simulink model "solar_collector_model_2019b"  (R2019b)
settings: Solver=VariableStepAuto  StartTime=0.0  StopTime=8760  FixedStep=1  RelTol=1e-3
values from neighbouring files (symbols this model uses):
  a1 = Ac*eta/C    (= 0.000575964912281)    [solar_collector_model_init.m]
  a2 = -UL_1*Ac/C    (= -0.00290974481659)    [solar_collector_model_init.m]
  a3 = -UL_2*Ac/C    (= -7.48006379585e-06)    [solar_collector_model_init.m]
  a4 = V^-1    (= 333.333333333)    [solar_collector_model_init.m]
  a5 = -a4    (= -333.333333333)    [solar_collector_model_init.m]
libraries: simulink x1
settings Model: Creator=Mariana  LastModifiedBy=admin

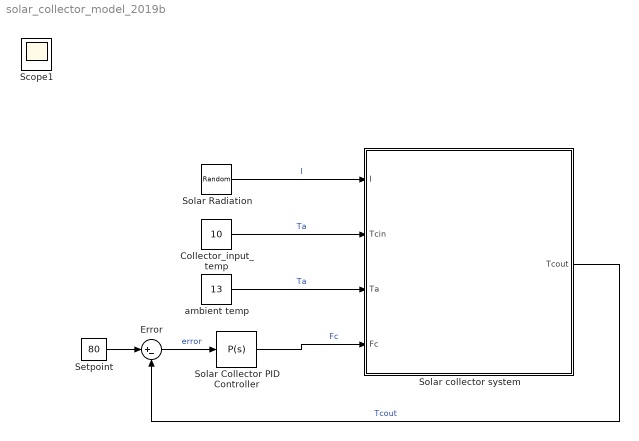
== system solar_collector_model_2019b ==
  "Collector_input_temp " : Constant  Value=10
  Error : Sum  Inputs=|+-
  Setpoint : Constant  Value=80
  Solar Collector PID Controller : simulink/Continuous/PID Controller  Controller=P  Form=Parallel  TimeDomain=Continuous-time  SampleTime=-1  IntegratorMethod=Forward Euler  FilterMethod=Forward Euler  ControllerParametersSource=internal  P=-0.0002  I=1.2  D=0.01  UseFilter=on  N=100  TunerSelectOption=Transfer Function Based (PID Tuner App)  ZeroCross=off  InitialConditionSource=internal  InitialConditionForIntegrator=0  InitialConditionForFilter=0  DifferentiatorICPrevScaledInput=0  ExternalReset=none  TrackingMode=off  Kt=1  LimitOutput=on  UpperSaturationLimit=0.00015  LowerSaturationLimit=0  LinearizeAsGain=on  AntiWindupMode=none  Kb=1  POutMin=[]  POutMax=[]  IOutMin=[]  IOutMax=[]  DOutMin=[]  DOutMax=[]  NOutMin=[]  NOutMax=[]  SumOutMin=[]  SumOutMax=[]  SaturationOutMin=[]  SaturationOutMax=[]  PParamMin=[]  PParamMax=[]  IParamMin=[]  IParamMax=[]  DParamMin=[]  DParamMax=[]  NParamMin=[]  NParamMax=[]  KbParamMin=[]  KbParamMax=[]  KtParamMin=[]  KtParamMax=[]  KbOutMin=[]  KbOutMax=[]  KtOutMin=[]  KtOutMax=[]  IntegratorOutMin=[]  IntegratorOutMax=[]  FilterOutMin=[]  FilterOutMax=[]  SumI1OutMin=[]  SumI1OutMax=[]  SumI2OutMin=[]  SumI2OutMax=[]  SumI3OutMin=[]  SumI3OutMax=[]  SumI4OutMin=[]  SumI4OutMax=[]  SumDOutMin=[]  SumDOutMax=[]  DifferentiatorOutMin=[]  DifferentiatorOutMax=[]  FilterDiffOutCoefMin=[]  FilterDiffOutCoefMax=[]  ReciprocalOutMin=[]  ReciprocalOutMax=[]  SumDenOutMin=[]  SumDenOutMax=[]  SumNumOutMin=[]  SumNumOutMax=[]  DivideOutMin=[]  DivideOutMax=[]  IntegratorContinuousStateAttributes=''  IntegratorStateMustResolveToSignalObject=off  IntegratorRTWStateStorageClass=Auto  FilterContinuousStateAttributes=''  FilterStateMustResolveToSignalObject=off  FilterRTWStateStorageClass=Auto  ParallelPVariant=InternalParameters  IdealPVariant=Disabled  IVariant=Disabled  DVariant=Disabled  IntegratorVariant=Disabled  SatVariant=Enabled  AWVariant=Disabled  PCopyVariant=Disabled  TRVariant=Disabled  FdbkBlocksVariant=Forward  IdealPFdbkVariant=Disabled  SatFdbkVariant=Disabled  DerivativeFilterVariant=Disabled  NVariant=Disabled  NCopyVariant=Disabled_SignalSpec  FilterICVariant=Disabled  IntegratorICVariant=Disabled  ExternalResetVariant=Disabled  TRSumVariant=Passthrough  SumFdbkVariant=Disabled  SumVariant=Passthrough_P
  Solar Radiation : RandomNumber  Mean=1200  Variance=0.5  SampleTime=0.1
  "Solar collector system " : Subsystem
      mask Display: image('collector_image.jpg'); % Use "Edit Image" on toolstrip to change.
  ambient temp : Constant  Value=13
  Scope1 : Scope
  wires:
  ambient temp/1 -> "Solar collector system "/3(Ta)  "Ta"
  Solar Radiation/1 -> "Solar collector system "/1(I)  "I"
  "Collector_input_temp "/1 -> "Solar collector system "/2(Tcin)  "Ta"
  Setpoint/1 -> Error/1
  "Solar collector system "/1(Tcout) -> Error/2  "Tcout"
  Error/1 -> Solar Collector PID Controller/1  "error"
  Solar Collector PID Controller/1 -> "Solar collector system "/4(Fc)  "Fc"

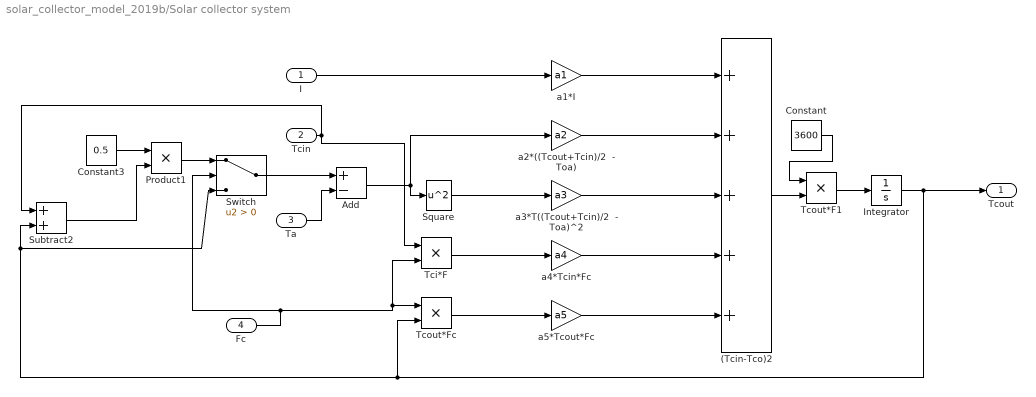
== system solar_collector_model_2019b/Solar collector system  ==
  I : Inport
  Tcin : Inport  Port=2
  Ta : Inport  Port=3
  Fc : Inport  Port=4
  (Tcin-Tco)2 : Sum  Inputs=+++++
  Add : Sum  Inputs=+-
  Constant : Constant  Value=3600
  Constant3 : Constant  Value=0.5
  Integrator : Integrator  InitialCondition=7.5
  Product1 : Product
  Square : Math  Operator=square  SignedPower=off  SaturateOnIntegerOverflow=on
  Subtract2 : Sum
  Switch : Switch  Criteria=u2 > Threshold  ZeroCross=off
  Tci*F : Product  Inputs=**
  Tcout*F1 : Product  Inputs=**
  Tcout*Fc : Product  Inputs=**
  a1*I : Gain  Gain=a1
  a2*((Tcout+Tcin)/2  - Toa) : Gain  Gain=a2
  a3*T((Tcout+Tcin)/2  - Toa)^2 : Gain  Gain=a3
  a4*Tcin*Fc : Gain  Gain=a4
  "a5*Tcout*Fc " : Gain  Gain=a5
  Tcout : Outport
  wires:
  a1*I/1 -> (Tcin-Tco)2/1
  Product1/1 -> Switch/1
  Switch/1 -> Add/1
  Subtract2/1 -> Product1/2
  Integrator/1 -> Tcout/1, Subtract2/2, Switch/3, Tcout*Fc/2
  Tcout*F1/1 -> Integrator/1
  Constant/1 -> Tcout*F1/1
  (Tcin-Tco)2/1 -> Tcout*F1/2
  Square/1 -> a3*T((Tcout+Tcin)/2  - Toa)^2/1
  Add/1 -> a2*((Tcout+Tcin)/2  - Toa)/1, Square/1
  Ta/1 -> Add/2
  I/1 -> a1*I/1
  "a5*Tcout*Fc "/1 -> (Tcin-Tco)2/5
  Fc/1 -> Switch/2, Tci*F/2, Tcout*Fc/1
  Tcout*Fc/1 -> "a5*Tcout*Fc "/1
  a4*Tcin*Fc/1 -> (Tcin-Tco)2/4
  Tci*F/1 -> a4*Tcin*Fc/1
  Tcin/1 -> Subtract2/1, Tci*F/1
  a2*((Tcout+Tcin)/2  - Toa)/1 -> (Tcin-Tco)2/2
  a3*T((Tcout+Tcin)/2  - Toa)^2/1 -> (Tcin-Tco)2/3
  Constant3/1 -> Product1/1
